simulink model "BallastResistor"  (R2025b)
settings: Solver=FixedStepAuto  StartTime=0.0  StopTime=100.0  FixedStep=Ts  RelTol=1e-3
values from neighbouring files (symbols this model uses):
  b_const = 1.0    (= 1)    [constants.m]
  ballast_fun_acceleration = 5    [constants.m]
  ballast_fun_deceleration = 5    [constants.m]
  fan_abs_delta = abs(fan_max_factor - fan_min_factor)    [constants.m]
  fan_max_factor = 1    [constants.m]
  fan_min_factor = 0.4    [constants.m]
  k_rad_ballast = 100.0    (= 100)    [constants.m]
  P_ballast_nom = 400000.0    (= 400000)    [constants.m]
  T_amb = 25.0    (= 25)    [constants.m]
  tau_ballast = 600.0    (= 600)    [constants.m]
  Ts = 0.001    [constants.m]
settings Model: TunableVars=J_AD,J_ICE,M_AD_nom,P_ballast_nom,P_oil_max,P_oil_min,T_AD_max,T_amb,T_ballast_max,T_cool_max,a_const,ad_fun_acceleration,b_const,k_heat,k_loss,k_loss0,k_rad_AD,k_rad_ballast,k_radiator,omega_ICE_max_prir,omega_ICE_max_run,tau,tau_AD_base,tau_ballast,tau_cool  TunableVarsStorageClass=Auto,Auto,Auto,Auto,Auto,Auto,Auto,Auto,Auto,Auto,Auto,Auto,Auto,Auto,Auto,Auto,Auto,Auto,Auto,Auto,Auto,Auto,Auto,Auto,Auto  TunableVarsTypeQualifier=,,,,,,,,,,,,,,,,,,,,,,,,  Creator=user  LastModifiedBy=user
settings OptimizationCC: DefaultParameterBehavior=Inlined  UseDivisionForNetSlopeComputation=on  GainParamInheritBuiltInType=on  UseFloatMulNetSlope=on  StrengthReduction=on  PassReuseOutputArgsAs=Individual arguments  NoFixptDivByZeroProtection=on  EfficientFloat2IntCast=on  OptimizeBlockOrder=speed  OptimizationPriority=Speed  OptimizationCustomize=off  MultiThreadedLoops=on  AutoScheduleForLoops=on  EfficientTunableParamExpr=on
settings DebuggingCC: ParameterTunabilityLossMsg=error
settings HardwareCC: ProdBitPerLong=64.0  ProdLongLongMode=on  ProdHWDeviceType=Intel->x86-64 (Linux 64)
settings SFSimCC: MATLABDynamicMemAlloc=off  SimTargetLang=C++  SimDLTargetLibrary=mkl-dnn
settings RTWCC: SystemTargetFile=ert.tlc  GenCodeOnly=on  TemplateMakefile=ert_default_tmf  GenerateReport=on  BuildConfiguration=Faster Runs  LaunchReport=on  TargetLang=C++  Description=Embedded Coder
settings CodeAppCC: ForceParamTrailComments=on  IgnoreCustomStorageClasses=off  OperatorAnnotations=on  SimulinkDataObjDesc=on  SFDataObjDesc=on  CustomSymbolStrGlobalVar=rt$N$M  CustomSymbolStrType=$N$M  CustomSymbolStrFcn=$N$M$F  CustomSymbolStrMacro=$N$M  InsertBlockDesc=on
settings ERTTargetCC: InlinedParameterPlacement=Hierarchical  RootIOFormat=Structure reference  ERTCustomFileTemplate=example_file_process.tlc  TargetLangStandard=C++17 (ISO)  GenerateSampleERTMain=on  CodeInterfacePackaging=Reusable function  SupportContinuousTime=on

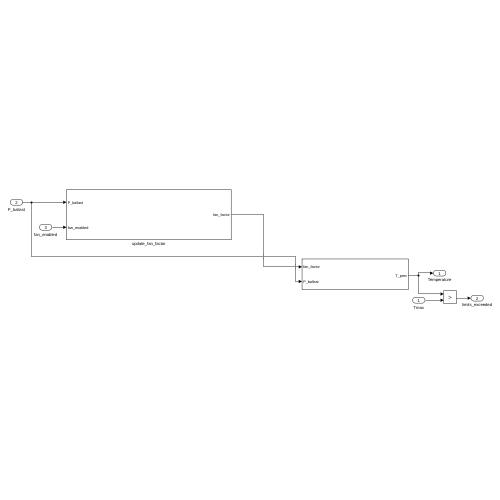
[thumbnail: Simulink's stored preview of the top-level diagram]
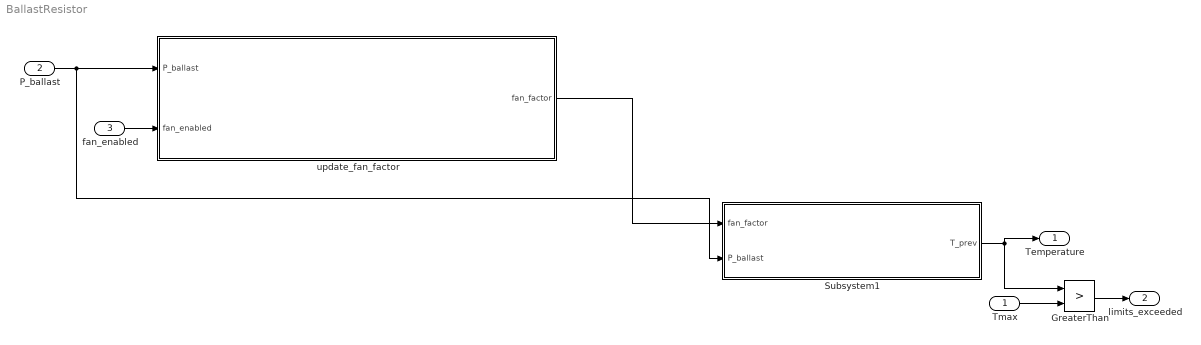
== system BallastResistor ==
  Tmax : Inport
  P_ballast : Inport  Port=2
  fan_enabled : Inport  Port=3
  GreaterThan : RelationalOperator  Operator=>  OutDataTypeStr=boolean  RndMeth=Simplest  InputSameDT=off
  Subsystem1 : Subsystem
  update_fan_factor : Subsystem
  Temperature : Outport
  limits_exceeded : Outport  Port=2
  wires:
  P_ballast/1 -> update_fan_factor/1(P_ballast), Subsystem1/2(P_ballast)
  fan_enabled/1 -> update_fan_factor/2(fan_enabled)
  update_fan_factor/1(fan_factor) -> Subsystem1/1(fan_factor)
  Subsystem1/1(T_prev) -> Temperature/1, GreaterThan/1
  Tmax/1 -> GreaterThan/2
  GreaterThan/1 -> limits_exceeded/1

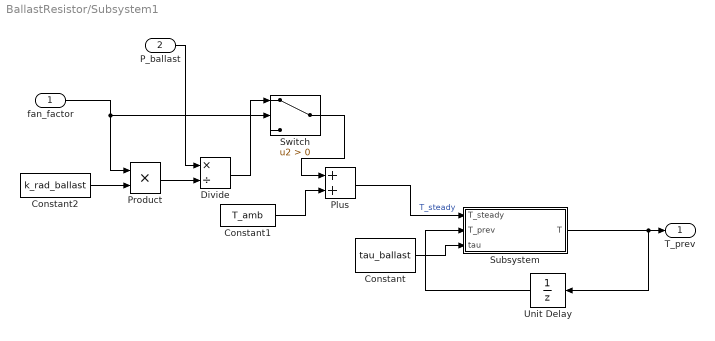
== system BallastResistor/Subsystem1 ==
  fan_factor : Inport
  P_ballast : Inport  Port=2
  Constant : Constant  Value=tau_ballast
  Constant1 : Constant  Value=T_amb
  Constant2 : Constant  Value=k_rad_ballast
  Divide : Product  Inputs=*/
  Plus : Sum
  Product : Product
  Subsystem : Subsystem
  Switch : Switch  Criteria=u2 > Threshold  SaturateOnIntegerOverflow=off  InputSameDT=off
  Unit Delay : UnitDelay  InitialCondition=T_amb  SampleTime=-1  HasFrameUpgradeWarning=on
  T_prev : Outport
  wires:
  Constant1/1 -> Plus/2
  Plus/1 -> Subsystem/1(T_steady)  "T_steady"
  Product/1 -> Divide/2
  Subsystem/1(T) -> Unit Delay/1, T_prev/1
  Constant2/1 -> Product/2
  fan_factor/1 -> Switch/2, Product/1
  P_ballast/1 -> Divide/1
  Unit Delay/1 -> Subsystem/2(T_prev)
  Divide/1 -> Switch/1
  Switch/1 -> Plus/1
  Constant/1 -> Subsystem/3(tau)

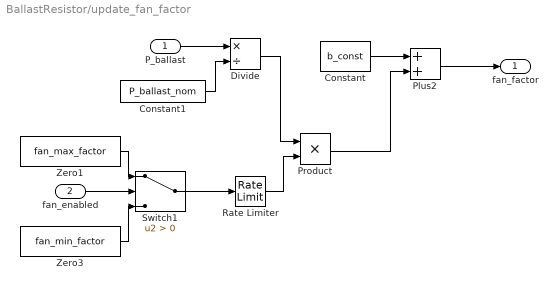
== system BallastResistor/update_fan_factor ==
  P_ballast : Inport
  fan_enabled : Inport  Port=2
  Constant : Constant  Value=b_const
  Constant1 : Constant  Value=P_ballast_nom
  Divide : Product  Inputs=*/
  Plus2 : Sum
  Product : Product
  Rate Limiter : RateLimiter  RisingSlewLimit=fan_abs_delta/ballast_fun_acceleration  FallingSlewLimit=-fan_abs_delta/ballast_fun_deceleration
  Switch1 : Switch  Criteria=u2 > Threshold  SaturateOnIntegerOverflow=off  InputSameDT=off
  Zero1 : Constant  Value=fan_max_factor  OutDataTypeStr=Inherit: Inherit via back propagation
  Zero3 : Constant  Value=fan_min_factor  OutDataTypeStr=Inherit: Inherit via back propagation
  fan_factor : Outport
  wires:
  P_ballast/1 -> Divide/1
  Zero3/1 -> Switch1/3
  Constant1/1 -> Divide/2
  Switch1/1 -> Rate Limiter/1
  Constant/1 -> Plus2/1
  fan_enabled/1 -> Switch1/2
  Plus2/1 -> fan_factor/1
  Zero1/1 -> Switch1/1
  Divide/1 -> Product/1
  Product/1 -> Plus2/2
  Rate Limiter/1 -> Product/2

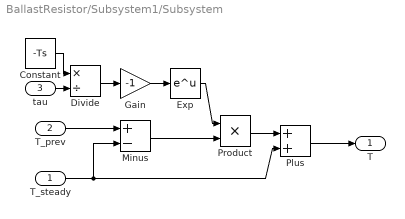
== system BallastResistor/Subsystem1/Subsystem ==
  T_steady : Inport
  T_prev : Inport  Port=2
  tau : Inport  Port=3
  Constant : Constant  Value=-Ts
  Divide : Product  Inputs=*/
  Exp : Math
  Gain : Gain  Gain=-1
  Minus : Sum  Inputs=+-
  Plus : Sum
  Product : Product
  T : Outport
  wires:
  T_prev/1 -> Minus/1
  T_steady/1 -> Plus/2, Minus/2
  Minus/1 -> Product/2
  Exp/1 -> Product/1
  Product/1 -> Plus/1
  Plus/1 -> T/1
  Divide/1 -> Gain/1
  Gain/1 -> Exp/1
  Constant/1 -> Divide/1
  tau/1 -> Divide/2
